simulink model "MCP_phase2_sineTrack_simulink"  (R2020a)
settings: Solver=VariableStepAuto  StartTime=0.0  StopTime=200  RelTol=1e-3
values from neighbouring files (symbols this model uses):
  A = double(Amat)    [MCP_phase2_linear.m]    (also in MCP_phase2_nonlinear.m)
  B = double(Bmat)    [MCP_phase2_linear.m]    (also in MCP_phase2_nonlinear.m)
  C = [1 0 0 0 0 0 ... (first row only)    [MCP_phase2_linear.m]    (also in MCP_phase2_nonlinear.m = [1 0 0 0)
  D = [0 0 ;0 0]    [MCP_phase2_linear.m]    (also in MCP_phase2_nonlinear.m = [0 0)
undefined symbols (not defined in the file or in its folder): a1, a2, b1, b2
settings Model: Creator=rafiee  LastModifiedBy=Lenovo
settings DataIOCC: ReturnWorkspaceOutputs=off
settings DebuggingCC: ArithmeticOperatorsInVariantConditions=warning
settings SFSimCC: SimUseLocalCustomCode=off  CustomCodeUndefinedFunction=UseInterfaceOnly
settings RTWCC: RTWUseLocalCustomCode=off
settings CodeAppCC: StateflowObjectComments=on

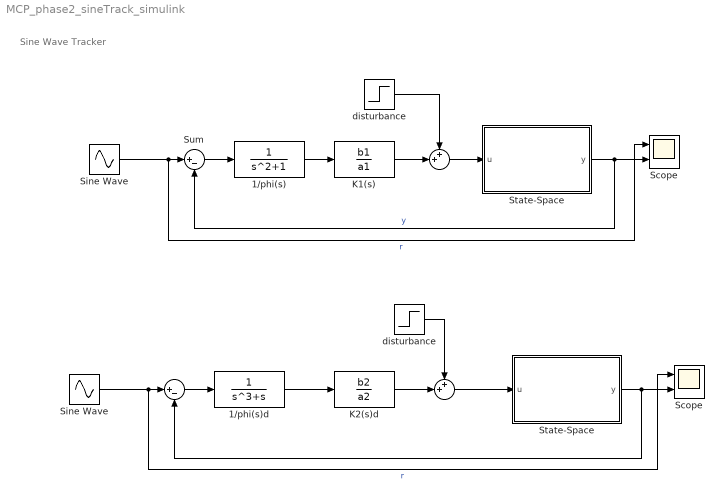
== system MCP_phase2_sineTrack_simulink ==
  note: Sine Wave Tracker
  " " : Sum  Inputs=|+-
  "  " : Sum  Inputs=++|
  "                       " : Sum  Inputs=++|
  1/phi(s) : TransferFcn  Denominator=[1 0 1]
  1/phi(s)d : TransferFcn  Denominator=[1 0 1 0]
  K1(s) : TransferFcn  Numerator=b1  Denominator=a1
  K2(s)d : TransferFcn  Numerator=b2  Denominator=a2
  Scope : Scope  NumInputPorts=2
  "Scope   " : Scope  NumInputPorts=2
  Sine Wave : Sin  SampleTime=0
  "Sine Wave " : Sin  SampleTime=0
  State-Space : Subsystem
  "State-Space " : Subsystem
  Sum : Sum  Inputs=|+-
  disturbance : Step  Time=30  After=20  SampleTime=0
  "disturbance " : Step  Time=30  After=2  SampleTime=0
  wires:
  1/phi(s)/1 -> K1(s)/1
  "State-Space "/1(y) -> Sum/2, Scope/2  "y"
  Sum/1 -> 1/phi(s)/1
  Sine Wave/1 -> Scope/1, Sum/1  "r"
  " "/1 -> 1/phi(s)d/1
  disturbance/1 -> "  "/1
  "Sine Wave "/1 -> " "/1, "Scope   "/1  "r"
  "  "/1 -> State-Space/1(u)
  State-Space/1(y) -> "Scope   "/2, " "/2
  K2(s)d/1 -> "  "/2
  1/phi(s)d/1 -> K2(s)d/1
  "                       "/1 -> "State-Space "/1(u)
  K1(s)/1 -> "                       "/2
  "disturbance "/1 -> "                       "/1

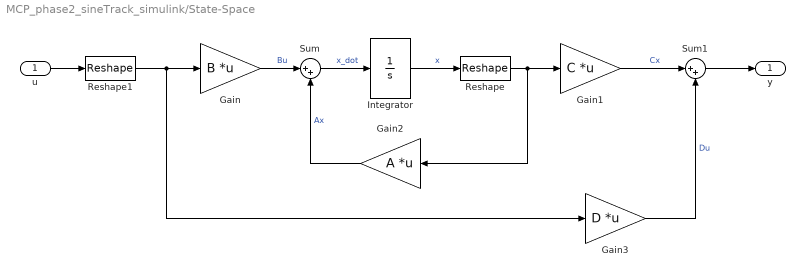
== system MCP_phase2_sineTrack_simulink/State-Space ==
  u : Inport
  Gain : Gain  Gain=B  Multiplication=Matrix(K*u)
  Gain1 : Gain  Gain=C  Multiplication=Matrix(K*u)
  Gain2 : Gain  Gain=A  Multiplication=Matrix(K*u)
  Gain3 : Gain  Gain=D  Multiplication=Matrix(K*u)
  Integrator : Integrator  InitialCondition=[0; 0; 0]
  Reshape : Reshape  OutputDimensionality=Column vector (2-D)  OutputDimensions=[12,1]
  Reshape1 : Reshape  OutputDimensionality=Column vector (2-D)
  Sum : Sum  Inputs=|++
  Sum1 : Sum  Inputs=|++
  y : Outport
  wires:
  Gain3/1 -> Sum1/2  "Du"
  Sum1/1 -> y/1
  u/1 -> Reshape1/1
  Reshape1/1 -> Gain/1, Gain3/1
  Reshape/1 -> Gain1/1, Gain2/1
  Gain2/1 -> Sum/2  "Ax"
  Gain1/1 -> Sum1/1  "Cx"
  Integrator/1 -> Reshape/1  "x"
  Sum/1 -> Integrator/1  "x_dot"
  Gain/1 -> Sum/1  "Bu"

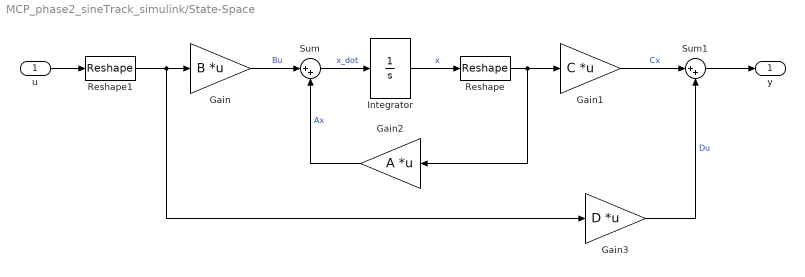
== system MCP_phase2_sineTrack_simulink/State-Space  ==
  u : Inport
  Gain : Gain  Gain=B  Multiplication=Matrix(K*u)
  Gain1 : Gain  Gain=C  Multiplication=Matrix(K*u)
  Gain2 : Gain  Gain=A  Multiplication=Matrix(K*u)
  Gain3 : Gain  Gain=D  Multiplication=Matrix(K*u)
  Integrator : Integrator  InitialCondition=[0; 0; 0]
  Reshape : Reshape  OutputDimensionality=Column vector (2-D)  OutputDimensions=[12,1]
  Reshape1 : Reshape  OutputDimensionality=Column vector (2-D)
  Sum : Sum  Inputs=|++
  Sum1 : Sum  Inputs=|++
  y : Outport
  wires:
  Gain/1 -> Sum/1  "Bu"
  Sum/1 -> Integrator/1  "x_dot"
  Integrator/1 -> Reshape/1  "x"
  Gain1/1 -> Sum1/1  "Cx"
  Gain2/1 -> Sum/2  "Ax"
  Reshape/1 -> Gain2/1, Gain1/1
  Reshape1/1 -> Gain3/1, Gain/1
  u/1 -> Reshape1/1
  Sum1/1 -> y/1
  Gain3/1 -> Sum1/2  "Du"
